simulink model "Lab1"  (Simulink 9.2)
settings: Solver=ode45  StartTime=0.0  StopTime=120  MaxStep=0.001  RelTol=1e-3  AbsTol=1e-6
settings Model: Creator=Shaocheng  LastModifiedBy=buddyugwumba1
settings SolverCC: AutoScaleAbsTol=off
settings DataIOCC: LimitDataPoints=off  Refine=4
settings OptimizationCC: BlockReduction=off  BooleanDataType=off  ExpressionDepthLimit=2147483647  InitFltsAndDblsToZero=on
settings DebuggingCC: SaveWithParameterizedLinksMsg=none  SignalResolutionControl=TryResolveAllWithWarning  MultiTaskDSMMsg=warning  MultiTaskCondExecSysMsg=none
settings HardwareCC: TargetUnknown=on
settings GRTTargetCC: TargetFcnLib=ansi_tfl_tmw.mat

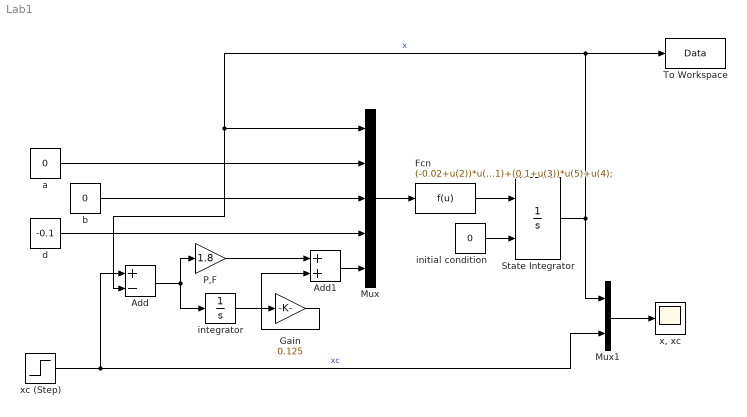
== system Lab1 ==
  Add : Sum  Inputs=+-
  Add1 : Sum
  Fcn : Fcn  Expr=(-0.02+u(2))*u(1)+(0.1+u(3))*u(5)+u(4);
  Gain : Gain  Gain=0.125
  Mux : Mux  Inputs=5
  Mux1 : Mux  Inputs=2
  P,F : Gain  Gain=1.8
  State Integrator : Integrator  InitialConditionSource=external
  To Workspace : ToWorkspace  VariableName=Data  SaveFormat=Structure With Time  SampleTime=-1
  a : Constant  Value=0
  b : Constant  Value=0
  d : Constant  Value=-0.1
  initial condition : Constant  Value=0
  integrator : Integrator
  "x, xc" : Scope
  xc (Step) : Step  Time=0  After=1.0  SampleTime=0
  wires:
  xc (Step)/1 -> Add/1, Mux1/2  "xc"
  State Integrator/1 -> Add/2, Mux/1, To Workspace/1, Mux1/1  "x"
  a/1 -> Mux/2
  b/1 -> Mux/3
  initial condition/1 -> State Integrator/2
  d/1 -> Mux/4
  Mux1/1 -> "x, xc"/1
  Add/1 -> P,F/1, integrator/1
  Add1/1 -> Mux/5
  P,F/1 -> Add1/1
  Mux/1 -> Fcn/1
  Fcn/1 -> State Integrator/1
  integrator/1 -> Gain/1
  Gain/1 -> Add1/2
